simulink model "rti1401_program_controls_2018"  (R2017b)
settings: Solver=ode1  StartTime=0.0  StopTime=Inf  FixedStep=0.001  RelTol=1e-3  EnableMultiTasking=on
PreLoadFcn:
  | dataCar
  | load_vars
  | structAero
  | structEstimPar
  | structSensors
  | structSettings
PostLoadFcn:
  | , if any(exist('dsrtsu_mdlpostloadfcn', 'file') == [2, 3, 6]), try dsrtsu_mdlpostloadfcn('Execute', bdroot); catch fprintf('Error in PostLoadFcn (dsrtsu_mdlpostloadfcn) for model "%s":\n %s\n', bdroot, lasterr); end, end,
InitFcn:
  | dataCar
  | load_vars
  | structAero
  | structEstimPar
  | structSensors
  | structSettings
StartFcn:
  | dataCar
  | load_vars
  | structAero
  | structEstimPar
  | structSensors
  | structSettings
values from neighbouring files (symbols this model uses):
  Throttle_limits = [0.15, 0.90, 0.16, 0.92]    [load_vars.m]
undefined symbols (not defined in the file or in its folder): car, sensors, tau
libraries: rtican x44, hdlsllib x32, simulink x8, rti1401lib_II_base x1
(part 10 of 11)

== system rti1401_program_controls_2018/Processor/Decisive Logic Block ==
  TorqueController : Inport
  rpmController : Inport  Port=2
  TorqueBypass : Inport  Port=3
  rpmBypass : Inport  Port=4
  Settings : Inport  Port=5
  MATLAB Function : MATLAB Function  TreatAsAtomicUnit=on
  Torques : Outport
  rpmRef : Outport  Port=2
  wires:
  TorqueController/1 -> MATLAB Function/1(torqueController)
  rpmController/1 -> MATLAB Function/2(rpmController)
  TorqueBypass/1 -> MATLAB Function/3(torqueBypass)
  rpmBypass/1 -> MATLAB Function/4(rpmBypass)
  MATLAB Function/2(rpmRef) -> rpmRef/1
  Settings/1 -> MATLAB Function/5(settings)
  MATLAB Function/1(torques) -> Torques/1

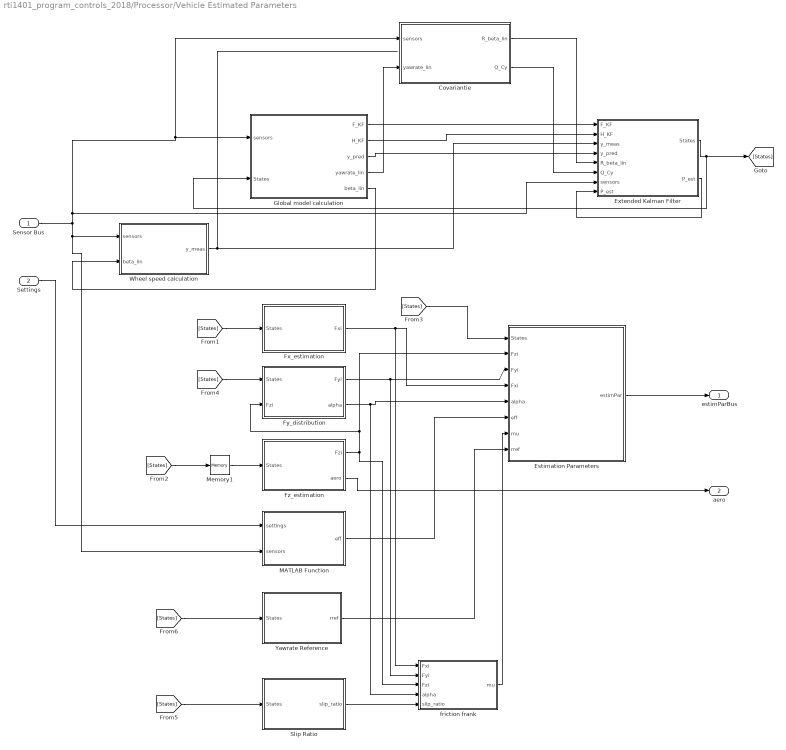
== system rti1401_program_controls_2018/Processor/Vehicle Estimated Parameters ==
  Sensor Bus : Inport
  Settings : Inport  Port=2
  Covariantie : MATLAB Function  TreatAsAtomicUnit=on
  Estimation Parameters : MATLAB Function  TreatAsAtomicUnit=on
  Extended Kalman Filter : MATLAB Function  TreatAsAtomicUnit=on
  Fx_estimation : MATLAB Function  TreatAsAtomicUnit=on
  Fy_distribution : MATLAB Function  TreatAsAtomicUnit=on
  Fz_estimation : MATLAB Function  TreatAsAtomicUnit=on
  Global model calculation : MATLAB Function  TreatAsAtomicUnit=on
  MATLAB Function : MATLAB Function  TreatAsAtomicUnit=on
  Memory1 : Memory
  Slip Ratio : MATLAB Function  TreatAsAtomicUnit=on
  Wheel speed calculation : MATLAB Function  TreatAsAtomicUnit=on
  Yawrate Reference : MATLAB Function  TreatAsAtomicUnit=on
  "friction frank  " : MATLAB Function  TreatAsAtomicUnit=on
  estimParBus : Outport
  aero : Outport  Port=2
  wires:
  Global model calculation/1(F_KF) -> Extended Kalman Filter/1(F_KF)
  Global model calculation/2(H_KF) -> Extended Kalman Filter/2(H_KF)
  Global model calculation/4(yawrate_lin) -> Covariantie/2(yawrate_lin)
  Wheel speed calculation/1(y_meas) -> Extended Kalman Filter/3(y_meas)
  Global model calculation/5(beta_lin) -> Wheel speed calculation/2(beta_lin)
  Covariantie/2(Q_Cy) -> Extended Kalman Filter/6(Q_Cy)
  Covariantie/1(R_beta_lin) -> Extended Kalman Filter/5(R_beta_lin)
  Extended Kalman Filter/1(States) -> [States], Global model calculation/2(States)
  Global model calculation/3(y_pred) -> Extended Kalman Filter/4(y_pred)
  Extended Kalman Filter/2(P_est) -> Extended Kalman Filter/8("P_est ")
  Estimation Parameters/1(estimPar) -> estimParBus/1
  [States] -> Fx_estimation/1(States)
  Memory1/1 -> Fz_estimation/1(States)
  [States] -> Memory1/1
  [States] -> Estimation Parameters/1(States)
  Fx_estimation/1(Fxi) -> "friction frank  "/1(Fxi), Estimation Parameters/4(Fxi)
  Fy_distribution/1(Fyi) -> "friction frank  "/2(Fyi), Estimation Parameters/3(Fyi)
  Fy_distribution/2(alpha) -> "friction frank  "/4(alpha), Estimation Parameters/5(alpha)
  [States] -> Fy_distribution/1(States)
  Fz_estimation/1(Fzi) -> "friction frank  "/3(Fzi), Fy_distribution/2(Fzi), Estimation Parameters/2(Fzi)
  Settings/1 -> MATLAB Function/1(settings)
  MATLAB Function/1(eff) -> Estimation Parameters/6(eff)
  Sensor Bus/1 -> Extended Kalman Filter/7(sensors), Covariantie/1(sensors), Global model calculation/1(sensors), MATLAB Function/2(sensors), Wheel speed calculation/1(sensors)
  "friction frank  "/1(mu) -> Estimation Parameters/7(mu)
  Slip Ratio/1(slip_ratio) -> "friction frank  "/5(slip_ratio)
  [States] -> Slip Ratio/1(States)
  Fz_estimation/2(aero) -> aero/1
  [States] -> Yawrate Reference/1(States)
  Yawrate Reference/1(rref) -> Estimation Parameters/8(rref)

== system rti1401_program_controls_2018/RTI Data/RTI Data Store ==
  RTI Data Store : Subsystem  mask(RTI_DATA_STORE){}
      mask help:
      | RTI Data Store Block. This block is used by RTI to store internal model dependent data. Deleting this block will result in data loss.
      |
      | NEVER DELETE, COPY, OR MODIFY THIS BLOCK!
      mask Help:
      | RTI Data Store Block. This block is used by RTI to store internal model dependent data. Deleting this block will result in data loss.
      | 
      | NEVER DELETE, COPY, OR MODIFY THIS BLOCK!
      mask Display: text(0.5, 0.5, ' ', 'HorizontalAlignment', 'center');

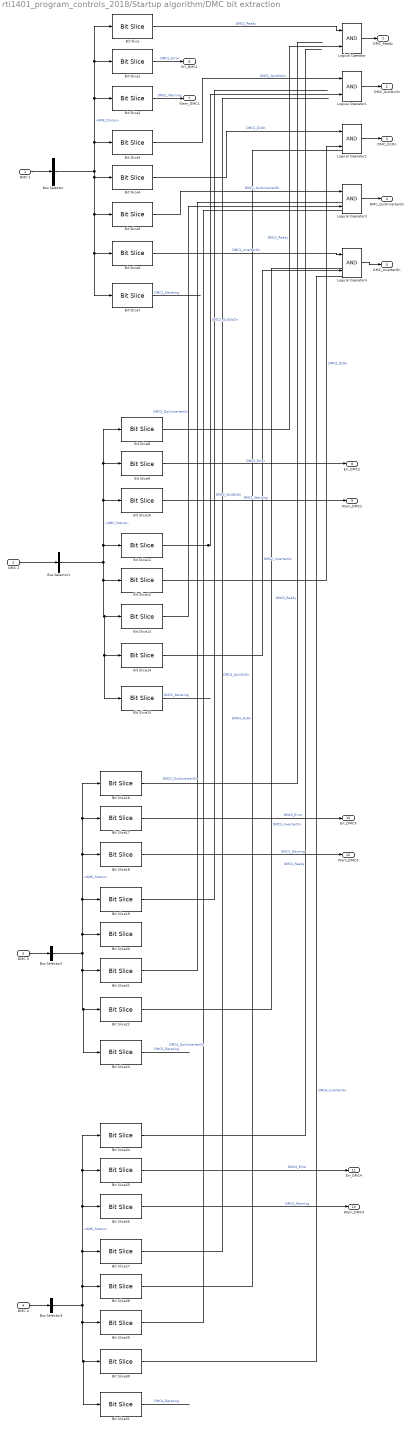
== system rti1401_program_controls_2018/Startup algorithm/DMC bit extraction ==
  DMC 1 : Inport
  DMC 2 : Inport  Port=2
  DMC 3 : Inport  Port=3
  DMC 4 : Inport  Port=4
  Bit Slice{,8,16,24} (4 alike) : hdlsllib/Logic and Bit Operations/Bit Slice  lidx=8  ridx=8
  Bit Slice{1,9,17,25} (4 alike) : hdlsllib/Logic and Bit Operations/Bit Slice  lidx=9  ridx=9
  Bit Slice{2,10,18,26} (4 alike) : hdlsllib/Logic and Bit Operations/Bit Slice  lidx=10  ridx=10
  Bit Slice{3,11,19,27} (4 alike) : hdlsllib/Logic and Bit Operations/Bit Slice  lidx=11  ridx=11
  Bit Slice{4,12,20,28} (4 alike) : hdlsllib/Logic and Bit Operations/Bit Slice  lidx=12  ridx=12
  Bit Slice{5,13,21,29} (4 alike) : hdlsllib/Logic and Bit Operations/Bit Slice  lidx=13  ridx=13
  Bit Slice{6,14,22,30} (4 alike) : hdlsllib/Logic and Bit Operations/Bit Slice  lidx=14  ridx=14
  Bit Slice{7,15,23,31} (4 alike) : hdlsllib/Logic and Bit Operations/Bit Slice  lidx=15  ridx=15
  Bus Selector{,1..3} (4 alike) : BusSelector  OutputSignals=AMK_Status
  Logical Operator{,1..4} (5 alike) : Logic  AllPortsSameDT=off  OutDataTypeStr=boolean
  DMC_Ready : Outport
  DMC_QuitDcOn : Outport  Port=2
  DMC_DcOn : Outport  Port=3
  DMC_QuitInverterOn : Outport  Port=4
  DMC_InverterOn : Outport  Port=5
  Err_DMC1 : Outport  Port=6
  Warn_DMC1 : Outport  Port=7
  Err_DMC2 : Outport  Port=8
  Warn_DMC2 : Outport  Port=9
  Err_DMC3 : Outport  Port=10
  Err_DMC4 : Outport  Port=11
  Warn_DMC3 : Outport  Port=12
  Warn_DMC4 : Outport  Port=13
  wires:
  DMC 4/1 -> Bus Selector3/1
  DMC 3/1 -> Bus Selector2/1
  DMC 1/1 -> Bus Selector/1
  DMC 2/1 -> Bus Selector1/1
  Bus Selector/1 -> Bit Slice7/1, Bit Slice6/1, Bit Slice5/1, Bit Slice4/1, Bit Slice/1, Bit Slice1/1, Bit Slice2/1, Bit Slice3/1  "<AMK_Status>"
  Bit Slice/1 -> Logical Operator/1  "DMC1_Ready"
  Bit Slice1/1 -> Err_DMC1/1  "DMC1_Error"
  Bit Slice2/1 -> Warn_DMC1/1  "DMC1_Warning"
  Bit Slice3/1 -> Logical Operator1/1  "DMC1_QuitDcOn"
  Bit Slice4/1 -> Logical Operator2/1  "DMC1_DcOn"
  Bit Slice5/1 -> Logical Operator3/1  "DMC1_QuitInverterOn"
  Bit Slice6/1 -> Logical Operator4/1  "DMC1_InverterOn"
  Bit Slice7/1 -> ?  "DMC1_Derating"
  Bus Selector1/1 -> Bit Slice15/1, Bit Slice14/1, Bit Slice13/1, Bit Slice12/1, Bit Slice8/1, Bit Slice9/1, Bit Slice10/1, Bit Slice11/1  "<AMK_Status>"
  Bit Slice8/1 -> Logical Operator/2  "DMC2_Ready"
  Bit Slice9/1 -> Err_DMC2/1  "DMC2_Error"
  Bit Slice10/1 -> Warn_DMC2/1  "DMC2_Warning"
  Bit Slice11/1 -> Logical Operator1/2  "DMC2_QuitDcOn"
  Bit Slice12/1 -> Logical Operator2/2  "DMC2_DcOn"
  Bit Slice13/1 -> Logical Operator3/2  "DMC2_QuitInverterOn"
  Bit Slice14/1 -> Logical Operator4/2  "DMC2_InverterOn"
  Bit Slice15/1 -> ?  "DMC2_Derating"
  Bus Selector2/1 -> Bit Slice16/1, Bit Slice17/1, Bit Slice18/1, Bit Slice19/1, Bit Slice20/1, Bit Slice23/1, Bit Slice22/1, Bit Slice21/1  "<AMK_Status>"
  Bit Slice16/1 -> ?  "DMC3_Ready"
  Bit Slice17/1 -> Err_DMC3/1  "DMC3_Error"
  Bit Slice18/1 -> Warn_DMC3/1  "DMC3_Warning"
  Bit Slice19/1 -> ?  "DMC3_QuitDcOn"
  Bit Slice21/1 -> ?  "DMC3_QuitInverterOn"
  Bit Slice22/1 -> ?  "DMC3_InverterOn"
  Bit Slice23/1 -> ?  "DMC3_Derating"
  Bus Selector3/1 -> Bit Slice24/1, Bit Slice25/1, Bit Slice26/1, Bit Slice27/1, Bit Slice28/1, Bit Slice31/1, Bit Slice30/1, Bit Slice29/1  "<AMK_Status>"
  Bit Slice24/1 -> ?  "DMC4_Ready"
  Bit Slice25/1 -> Err_DMC4/1  "DMC4_Error"
  Bit Slice26/1 -> Warn_DMC4/1  "DMC4_Warning"
  Bit Slice27/1 -> ?  "DMC4_QuitDcOn"
  Bit Slice28/1 -> ?  "DMC4_DcOn"
  Bit Slice29/1 -> ?  "DMC4_QuitInverterOn"
  Bit Slice30/1 -> ?  "DMC4_InverterOn"
  Bit Slice31/1 -> ?  "DMC4_Derating"
  Logical Operator/1 -> DMC_Ready/1
  Logical Operator1/1 -> DMC_QuitDcOn/1
  Logical Operator2/1 -> DMC_DcOn/1
  Logical Operator3/1 -> DMC_QuitInverterOn/1
  Logical Operator4/1 -> DMC_InverterOn/1

== system rti1401_program_controls_2018/Startup algorithm/Merge_Controlword ==
  Control_in : Inport
  DcOn : Inport  Port=2
  Enable : Inport  Port=3
  InverterOn : Inport  Port=4
  ErrorReset : Inport  Port=5
  Bus Creator : BusCreator  Inputs=4
  If CTRL = Null : MATLAB Function  TreatAsAtomicUnit=on
  Control : Outport
  wires:
  Enable/1 -> If CTRL = Null/3(En_in)
  InverterOn/1 -> If CTRL = Null/4(Inv_in)
  DcOn/1 -> If CTRL = Null/2(Dc_in)
  Control_in/1 -> If CTRL = Null/1(Ctrl_in)
  If CTRL = Null/1(DcOn) -> Bus Creator/1
  If CTRL = Null/2(Enable) -> Bus Creator/2
  If CTRL = Null/3(InverterOn) -> Bus Creator/3
  Bus Creator/1 -> Control/1  "Controlbits"
  ErrorReset/1 -> Bus Creator/4  "ErrorReset"

== system rti1401_program_controls_2018/Processor/Control Systems/Distributor ==
  sensors : Inport
  settings : Inport  Port=2
  estimPar : Inport  Port=3
  Mz : Inport  Port=4
  Aero : Inport  Port=5
  MATLAB Function : MATLAB Function  TreatAsAtomicUnit=on
  Mux : Mux
  To Workspace : ToWorkspace  VariableName=Fdes  SaveFormat=Timeseries  SampleTime=-1
  To Workspace1 : ToWorkspace  VariableName=Fxmax  SaveFormat=Timeseries  SampleTime=-1
  To Workspace2 : ToWorkspace  VariableName=MdesFdesFxmaxFx  SaveFormat=Timeseries  SampleTime=-1
  To Workspace4 : ToWorkspace  VariableName=Fx  SaveFormat=Timeseries  SampleTime=-1
  Torque/Brake analyzer : Subsystem
  torqueDistribution : Outport
  slipSet : Outport  Port=2
  wires:
  MATLAB Function/1(torqueDistribution) -> torqueDistribution/1
  sensors/1 -> Torque/Brake analyzer/1(sensors), MATLAB Function/1(sensors)
  settings/1 -> Torque/Brake analyzer/2(settings), MATLAB Function/2(settings)
  estimPar/1 -> Torque/Brake analyzer/3(estimPar), MATLAB Function/3(estimPar)
  Mz/1 -> Mux/1, MATLAB Function/4(Mz)
  MATLAB Function/2(slipSet) -> slipSet/1
  MATLAB Function/3(Fdes) -> Mux/2, To Workspace/1
  Mux/1 -> To Workspace2/1
  MATLAB Function/5(Fx) -> To Workspace4/1, Mux/4
  MATLAB Function/4(Fxmax) -> To Workspace1/1, Mux/3
  Torque/Brake analyzer/1(Fdes) -> MATLAB Function/5("Fdes ")
  Aero/1 -> Torque/Brake analyzer/4(Aero)

== system rti1401_program_controls_2018/Processor/Control Systems/Power Checker ==
  Sensors : Inport
  Settings : Inport  Port=2
  "estimPar  " : Inport  Port=3
  unchecked torque : Inport  Port=4
  Power checker : MATLAB Function  TreatAsAtomicUnit=on
  CheckedTorque : Outport
  wires:
  Sensors/1 -> Power checker/1(sensors)
  Settings/1 -> Power checker/2(settings)
  Power checker/1(CheckedTorque) -> CheckedTorque/1
  "estimPar  "/1 -> Power checker/3(estimPar)
  unchecked torque/1 -> Power checker/4(UncheckedTorque)

== system rti1401_program_controls_2018/RTI Data/RTI Data Store/RTI Data Store ==
  RTI Data Store : Subsystem  mask(RTI_DATA_STORE){}
      mask help:
      | RTI Data Store Block. This block is used by RTI to store internal model dependent data. Deleting this block will result in data loss.
      |
      | NEVER DELETE, COPY, OR MODIFY THIS BLOCK!
      mask Help:
      | RTI Data Store Block. This block is used by RTI to store internal model dependent data. Deleting this block will result in data loss.
      | 
      | NEVER DELETE, COPY, OR MODIFY THIS BLOCK!
      mask Display: text(0.5, 0.5, ' ', 'HorizontalAlignment', 'center');

== system rti1401_program_controls_2018/Processor/Control Systems/Distributor/Torque//Brake analyzer ==
  sensors : Inport
  settings : Inport  Port=2
  estimPar : Inport  Port=3
  Aero : Inport  Port=4
  MATLAB Function1 : MATLAB Function  TreatAsAtomicUnit=on
  Fdes : Outport
  wires:
  MATLAB Function1/1(Fdes) -> Fdes/1
  sensors/1 -> MATLAB Function1/1(sensors)
  settings/1 -> MATLAB Function1/2(settings)
  estimPar/1 -> MATLAB Function1/3(estimPar)
  Aero/1 -> MATLAB Function1/4(aero)

== system rti1401_program_controls_2018/RTI Data/RTI Data Store/RTI Data Store/RTI Data Store ==
  RTI Data Store : Subsystem  mask(RTI_DATA_STORE){}
      mask help:
      | RTI Data Store Block. This block is used by RTI to store internal model dependent data. Deleting this block will result in data loss.
      |
      | NEVER DELETE, COPY, OR MODIFY THIS BLOCK!
      mask Help:
      | RTI Data Store Block. This block is used by RTI to store internal model dependent data. Deleting this block will result in data loss.
      | 
      | NEVER DELETE, COPY, OR MODIFY THIS BLOCK!
      mask Display: text(0.5, 0.5, ' ', 'HorizontalAlignment', 'center');

== system rti1401_program_controls_2018/RTI Data/RTI Data Store/RTI Data Store/RTI Data Store/RTI Data Store ==

== matlab function rti1401_program_controls_2018/Inputs/Preprocessor/MATLAB Function ==
  data: Throttle1 input; error output; Throttle2 input; limits input; throttle output
function [error,throttle]= ThrottleSensorPreprocessor(Throttle1, Throttle2, limits)
% Variables
lowerlim1 = limits(1);
upperlim1 = limits(2);
lowerlim2 = limits(3);
upperlim2 = limits(4);

% Throttle sensor 1

if Throttle1<lowerlim1
    y1=0;
elseif Throttle1>upperlim1
    y1=1;
else
   y1=Throttle1; %%schalen???
end

%Throttle sensor 2

if Throttle2<lowerlim2
    y2=0;
elseif Throttle2>upperlim2
    y2=1;
else
   y2=Throttle2; %%schalen???
end


% Error
if abs(Throttle1-Throttle2) > 0.10
    error = 1;
    throttle = 0;
else
    error = 0;
    throttle = double((y1+y2)/2);
end

== matlab function rti1401_program_controls_2018/Outputs/Splitter ==
  data: Torques input; torqueFL_Pos output; torqueFL_Neg output; wheelspeedFL output; torqueFR_Pos output; torqueFR_Neg output; wheelspeedFR output; torqueRL_Pos output; torqueRL_Neg output; wheelspeedRL output; torqueRR_Pos output; torqueRR_Neg output; wheelspeedRR output; status input; car parameter
function [torqueFL_Pos, torqueFL_Neg, wheelspeedFL, ...
    torqueFR_Pos, torqueFR_Neg, wheelspeedFR, ...
    torqueRL_Pos, torqueRL_Neg, wheelspeedRL, ...
    torqueRR_Pos, torqueRR_Neg, wheelspeedRR]= Splitter(Torques, status, car)

inversetorque = car.motor.Tmax;

if (status == 4)

    if Torques(1) >= 0
        torqueFL_Pos = int16(Torques(1)*1000);
        torqueFL_Neg = int16(-inversetorque(1)*1000);
        wheelspeedFL = int16(500);
    else
        torqueFL_Pos = int16(inversetorque(1)*1000);
        torqueFL_Neg = int16(Torques(1)*1000);
        wheelspeedFL = int16(0);
    end

    if Torques(2) >= 0
        torqueFR_Pos = int16(Torques(2)*1000);
        torqueFR_Neg = int16(-inversetorque(2)*1000);
        wheelspeedFR = int16(500);
    else
        torqueFR_Pos = int16(inversetorque(2)*1000);
        torqueFR_Neg = int16(Torques(2)*1000);
        wheelspeedFR = int16(0);
    end

    if Torques(3) >= 0
        torqueRL_Pos = int16(Torques(3)*1000);
        torqueRL_Neg = int16(-inversetorque(3)*1000);
        wheelspeedRL = int16(500);
    else
        torqueRL_Pos = int16(inversetorque(3)*1000);
        torqueRL_Neg = int16(Torques(3)*1000);
        wheelspeedRL = int16(0);
    end

    if Torques(4) >= 0
        torqueRR_Pos = int16(Torques(4)*1000);
        torqueRR_Neg = int16(-inversetorque(4)*1000);
        wheelspeedRR = int16(500);
    else
        torqueRR_Pos = int16(inversetorque(4)*1000);
        torqueRR_Neg = int16(Torques(4)*1000);
        wheelspeedRR = int16(0);
    end
else
    torqueFL_Pos = int16(0);
    torqueFL_Neg = int16(0);
    wheelspeedFL = int16(0);
    torqueFR_Pos = int16(0);
    torqueFR_Neg = int16(0);
    wheelspeedFR = int16(0);
    torqueRL_Pos = int16(0);
    torqueRL_Neg = int16(0);
    wheelspeedRL = int16(0);
    torqueRR_Pos = int16(0);
    torqueRR_Neg = int16(0);
    wheelspeedRR = int16(0);
end

== matlab function rti1401_program_controls_2018/Inputs/Preprocessor/Throttle1 perc ==
  data: u input; y output
function y = percentage(u)
y = ((1024 - double(u)) - 74) / 380;

== matlab function rti1401_program_controls_2018/Inputs/Preprocessor/Throttle2 perc off ==
  data: u input; y output
function y = percoff(u)
y = (1024 - double(u) - 374) / 420;

== matlab function rti1401_program_controls_2018/Inputs/Preprocessor/Acc conversion ==
  data: x input; y input; z input; AccX output; AccY output; AccZ output
function [AccX,AccY,AccZ] = AccConv(x,y,z)
AccX = x*9.81;
AccY = y*9.81;
AccZ = z*9.81;

== matlab function rti1401_program_controls_2018/Inputs/Preprocessor/YR//RR conversion ==
  data: y input; r input; Y output; R output
function [Y,R] = YRRR(y,r)
Y = y*10*2*pi;
R = r*10*2*pi;

== matlab function rti1401_program_controls_2018/Inputs/Preprocessor/Steering conv ==
  data: u input; Steering output
function Steering = steeringangle(u)
t = double(u);
Steering = 1 * t; %TODO: conversion factor, output = rack travel in mm

== matlab function rti1401_program_controls_2018/Inputs/EnergyMeter/parseCurrent  ==
  data: Mux input; current output; status input; messageNr input; valueHighest input; valueMidHigh input; valueMidLow input; valueLowest input
function current = value(Mux,status,messageNr,valueHighest,valueMidHigh, valueMidLow, valueLowest)
%    format hex;
   
  
    value = [valueLowest, valueMidLow, valueMidHigh, valueHighest];
    value = typecast(value, 'uint32');
    current=uint32(0);
    %0 is current
%     disp (Mux);
%     disp (status);
%     disp (messageNr);
%     disp (valueHigh);
%     disp (valueLow);
%     value = [valueHigh,valueLow];
%     disp (value);
    if Mux==0
        if status==0
            %status ok
            current = value %swapbytes(typecast(value,'uint32'));%current in mA
        else
        end
    end
%     disp (current);
%     format long;
%     disp (current);
end

== matlab function rti1401_program_controls_2018/Inputs/EnergyMeter/parseVoltage1 ==
  data: Mux input; voltage1 output; status input; messageNr input; valueHighest input; valueMidHigh input; valueMidLow input; valueLowest input
function voltage1 = value(Mux,status,messageNr,valueHighest,valueMidHigh,valueMidLow,valueLowest)
%    format hex;
    voltage1=uint32(0);
    %0 is current
%     disp (Mux);
%     disp (status);
%     disp (messageNr);
%     disp (valueHigh);
%     disp (valueLow);
    value = [valueLowest, valueMidLow, valueMidHigh, valueHighest];
    value = typecast(value, 'uint32');
%     disp (value);
    if Mux==1
        if status==0
            %status ok
            voltage1 = value;
        else
        end
    end
%     disp (current);
%     format long;
%     disp (current);
end

== matlab function rti1401_program_controls_2018/Inputs/EnergyMeter/parseVoltage3 ==
  data: Mux input; voltage3 output; status input; messageNr input; valueHighest input; valueMidHigh input; valueMidLow input; valueLowest input
function voltage3 = value(Mux,status,messageNr,valueHighest,valueMidHigh,valueMidLow,valueLowest)
%    format hex;
   
    voltage3=uint32(0);
    %0 is current
%     disp (Mux);
%     disp (status);
%     disp (messageNr);
%     disp (valueHigh);
%     disp (valueLow);
    value = [valueLowest, valueMidLow, valueMidHigh, valueHighest];
    value = typecast(value, 'uint32');
%     disp (value);
    if Mux==3
        if status==0
            %status ok
            voltage3 = value;
        else
        end
    end
%     disp (current);
%     format long;
%     disp (current);
end

== matlab function rti1401_program_controls_2018/Inputs/EnergyMeter/parseTemperature ==
  data: Mux input; temperature output; status input; messageNr input; valueHighest input; valueMidHigh input; valueMidLow input; valueLowest input
function temperature = value(Mux,status,messageNr,valueHighest,valueMidHigh,valueMidLow,valueLowest)
%    format hex;
    
    temperature=uint32(0);
    %0 is current
%     disp (Mux);
%     disp (status);
%     disp (messageNr);
%     disp (valueHigh);
%     disp (valueLow);
    value = [valueLowest, valueMidLow, valueMidHigh, valueHighest];
    value = typecast(value, 'uint32');
%     disp (value);
    if Mux==4
        if status==0
            %status ok
            temperature =value;
        else
        end
    end
%     disp (current);
%     format long;
%     disp (current);
end

== matlab function rti1401_program_controls_2018/Inputs/EnergyMeter/parseEnergy ==
  data: Mux input; energy output; status input; messageNr input; valueHighest input; valueMidHigh input; valueMidLow input; valueLowest input
function energy = value(Mux,status,messageNr,valueHighest,valueMidHigh,valueMidLow,valueLowest)
%    format hex;
    
    energy= uint32(0);
    %0 is current
%     disp (Mux);
%     disp (status);
%     disp (messageNr);
%     disp (valueHigh);
%     disp (valueLow);
    value = [valueLowest, valueMidLow, valueMidHigh, valueHighest];
    value = typecast(value, 'uint32');
%     disp (value);
    if Mux==5
        if status==0
            %status ok
            energy =value;
        else
        end
    end
%     disp (current);
%     format long;
%     disp (current);
end

== matlab function rti1401_program_controls_2018/Inputs/EnergyMeter/MATLAB Function ==
  data: muxByte input; response output; response0 input; response1 input; response2 input; response3 input; response4 input; response5 input; response6 input
function response = response(muxByte,response0, response1,response2,response3,response4,response5,response6)
    error = uint8(255);
    size = zeros(1,7);
    response = uint8(size);
    if (muxByte >= 128 && muxByte < 144)
       %error/log data
       if (muxByte < 130) % 0x82
          response(1) = error;
       end
       if (muxByte == 130||muxByte == 131) %response on overal logdata, 0x82 en 0x83
           response = [response0, response1, response2, response3, response4, response5, response6];
       end
    end
    if (muxByte >=144 && muxByte < 160)
       %can id 
       switch muxByte
           case 144
           case 145
           case 146
           case 147
           case 148
           case 149
           case 150
           case 151
           case 157
           case 159
           otherwise
               response(1) = error;
       end               
    end
    if (muxByte >=160 && muxByte < 176)
       %config result
       %cases zoals bij 90
       %default
       response(1) = error;
    end
    if (muxByte >=176 && muxByte < 192)
        %set en get commands
        %B0 - B6, B9 - BC
        response(1) = error;
    end
    if (muxByte == 255)
        response(1) = error;
    end
end

== matlab function rti1401_program_controls_2018/Setup/MATLAB Function ==
  data: messageByte0 output; messageByte1 output; messageByte2 output; messageByte3 output; messageByte4 output; messageByte5 output; messageByte6 output; messageByte7 output; progress output; initialProgress input
function [messageByte0,messageByte1,messageByte2,messageByte3, messageByte4, messageByte5, messageByte6,messageByte7,progress] = setup(initialProgress)
    progress = initialProgress;
    messageValue = uint8(zeros(1,8));
    if (progress<5)
        if(progress==0)
            messageValue(1) = uint8(52); %0x34 set_mode --> stop
            messageValue(2:8)= uint8(zeros(1,7));
            progress=1;
        elseif(progress==1)
            messageValue(1) = uint8(33); %0x21 set configuration of U1
            messageValue(2) = uint8(2); %0x02 cyclisch && big endian
            messageValue(3:4) = uint8([0 50]); %50ms 
            messageValue(5:8) = zeros(1,4);
            progress=2;
        elseif(progress==2)
            messageValue(1) = uint8(37); %0x25 set configuration of W
            messageValue(2) = uint8(2); %0x02 cyclisch && big endian
            messageValue(3:4) = uint8([0 50]); %50ms 
            messageValue(5:8) = zeros(1,4);
            progress = 3;
        elseif(progress ==3)
            messageValue(1) = uint8(38); %0x26 set configuration of As
            messageValue(2) = uint8(2); %0x02 cyclisch && big endian
            messageValue(3:4) = uint8([0 50]); %50ms 
            messageValue(5:8) = zeros(1,4);
            progress = 4;
        elseif (progress ==4)
            messageValue(1) = uint8(52); %0x34 set_mode--> start
            messageValue(2:3) = uint8(ones(1,2));
            messageValue(4:8) = zeros(1,5);
            progress=5;
        end
    end
    messageByte0 = messageValue(1);
    messageByte1 = messageValue(2);
    messageByte2 = messageValue(3);
    messageByte3 = messageValue(4);
    messageByte4 = messageValue(5);
    messageByte5 = messageValue(6);
    messageByte6 = messageValue(7);
    messageByte7 = messageValue(8);
end

== matlab function rti1401_program_controls_2018/Processor/Lode Torque Conversion Block ==
  data: currentFL input; torqueFL output; currentFR input; currentRL input; currentRR input; torqueFR output; torqueRL output; torqueRR output
function [torqueFL,torqueFR,torqueRL,torqueRR] = torqueConversion(currentFL,currentFR,currentRL,currentRR)
currentFL = double(currentFL);
currentFR = double(currentFR);
currentRL = double(currentRL);
currentRR = double(currentRR);

ID110 = 107.2; %Converter peak current (from Ipex Pro)

%4.1837 = Nominal Current/Nominal Torque = 41A/9.8Nm (from AMK data sheet)
%--> Ook geldig voor anno 2018!!

IqFL = currentFL * ID110 / 16384; %I_q (AMK manual P65)
torqueFL = IqFL / 4.1837; %T (AMK manual P65)

IqFR = currentFR * ID110 / 16384; %I_q (AMK manual P65)
torqueFR = IqFR / 4.1837; %T (AMK manual P65)

IqRL = currentRL * ID110 / 16384; %I_q (AMK manual P65)
torqueRL = IqRL / 4.1837; %T (AMK manual P65)

IqRR = currentRR * ID110 / 16384; %I_q (AMK manual P65)
torqueRR = IqRR / 4.1837; %T (AMK manual P65)

== matlab function rti1401_program_controls_2018/Inputs/EnergyMeter/parseVoltage2 ==
  data: Mux input; voltage2 output; status input; messageNr input; valueHighest input; valueMidHigh input; valueMidLow input; valueLowest input
function voltage2 = value(Mux,status,messageNr,valueHighest,valueMidHigh,valueMidLow,valueLowest)
%    format hex;
    
    voltage2=uint32(0);
    %0 is current
%     disp (Mux);
%     disp (status);
%     disp (messageNr);
%     disp (valueHigh);
%     disp (valueLow);
    value = [valueLowest, valueMidLow, valueMidHigh, valueHighest];
    value = typecast(value, 'uint32');
%     disp (value);
    if Mux==2
        if status==0
            %status ok
            voltage2 = value;
        else
        end
    end
%     disp (current);
%     format long;
%     disp (current);
end

== matlab function rti1401_program_controls_2018/Inputs/EnergyMeter/parseAs ==
  data: Mux input; ampereSeconde output; status input; messageNr input; valueHighest input; valueMidHigh input; valueMidLow input; valueLowest input
function ampereSeconde = value(Mux,status,messageNr,valueHighest,valueMidHigh,valueMidLow,valueLowest)
%    format hex;
    ampereSeconde=uint32(6);
    %0 is current
%     disp (Mux);
%     disp (status);
%     disp (messageNr);
%     disp (valueHigh);
%     disp (valueLow);
    value = [valueLowest, valueMidLow, valueMidHigh, valueHighest];
    value = typecast(value, 'uint32');
%     disp (value);
    if Mux==3
        if status==0
            %status ok
            ampereSeconde = value;
        else
        end
    end
%     disp (current);
%     format long;
%     disp (current);
end

== matlab function rti1401_program_controls_2018/Inputs/EnergyMeter/parseWh ==
  data: Mux input; wattHour output; status input; messageNr input; valueHighest input; valueMidHigh input; valueMidLow input; valueLowest input
function wattHour = value(Mux,status,messageNr,valueHighest,valueMidHigh,valueMidLow,valueLowest)
%    format hex;
 
    wattHour=uint32(0);
    %0 is current
%     disp (Mux);
%     disp (status);
%     disp (messageNr);
%     disp (valueHigh);
%     disp (valueLow);
    value = [valueLowest, valueMidLow, valueMidHigh, valueHighest];
    value = typecast(value, 'uint32');
%     disp (value);
    if Mux==7
        if status==0
            %status ok
            wattHour = value;
        else
        end
    end
%     disp (current);
%     format long;
%     disp (current);
end

== stateflow chart rti1401_program_controls_2018/Startup algorithm/Startup ==
  state LVOn
    entry: AMK_Control = 1;
    entry: BMS_START= 1;
    entry: AMK_DcOn = 0;
    entry: AMK_Enable = 0;
    entry: AMK_InverterOn = 0;
    entry: Status = 0;
  state SystemReady
    entry: BMS_START = 1;
    entry: Status = 1;
  state SwitchDCOn
    entry: Status = 2;
    entry: AMK_DcOn = 1;
  state PreparingToDrive
    entry: AMK_Enable = 1;
    entry: AMK_InverterOn = 1;
    entry: RTDS = true;
    entry: Status = 3;
  state Running
    entry: Status = 4;
    entry: RTDS = false;
  SystemReady -> LVOn [order 2] : [Stop==1]
  (default) -> LVOn
  LVOn -> SystemReady : [AMK_Systemready == 1 && Stop==0]
  Running -> LVOn : [Stop == 1]
  SystemReady -> SwitchDCOn [order 1] : [Start==1]
  PreparingToDrive -> LVOn [order 2] : [Stop ==1]
  SwitchDCOn -> LVOn [order 2] : [Stop == 1]
  SwitchDCOn -> PreparingToDrive [order 1] : [QuitDcOn==1 && DcOn==1]
  PreparingToDrive -> Running [order 1] : [InverterOn==1 && QuitInverterOn==1]
  data: AMK_Systemready input; BMS_HV input; AMK_Control output; AMK_DcOn output; AMK_Enable output; AMK_InverterOn output; BMS_START output; RTDS output; Status output; QuitDcOn input; DcOn input; InverterOn input; QuitInverterOn input; Start input; Stop input

== matlab function rti1401_program_controls_2018/Inputs/Preprocessor/Brake 1 perc  ==
  data: u input; y output
function y = percentage(u)
y = u/65536;

== matlab function rti1401_program_controls_2018/Inputs/Preprocessor/Brake 2 perc  ==
  data: u input; y output
function y = percentage(u)
y = u/65536;

== matlab function rti1401_program_controls_2018/Startup algorithm/Merge_Controlword/If CTRL = Null ==
  data: Ctrl_in input; DcOn output; Dc_in input; En_in input; Inv_in input; Enable output; InverterOn output
function [DcOn, Enable, InverterOn] = fcn(Ctrl_in, Dc_in, En_in, Inv_in)
%#codegen

if (Ctrl_in==0)
    DcOn = false;
    Enable = false;
    InverterOn = false;
else
    DcOn = logical(Dc_in);
    Enable = logical(En_in);
    InverterOn = logical(Inv_in);
end

== matlab function rti1401_program_controls_2018/Processor/Breyne Pedal Mapping ==
  data: throttle input; throttle_out output; regen input; brake_out output
function [throttle_out, brake_out] = pedalmapping(throttle, regen)

%Pedal mapping: partially regenarative braking (parabolic), partially positive 
%power (parabolic and linear)
%IMPORTANT: D = shape factor = relative y-value where parabolic switches to linear
% (between 0 and 1)
% LOW D = more linear
% HIGH D = more parabolic

D = double(0);

%%
regen = double(max(min(regen,30),0));
throttle_acc = double((throttle-regen)/(100-regen));
if throttle >= regen
    if throttle <= regen+(100-regen)*(2*D)/(1+D)
        if throttle == regen %iow if D==0
            throttle_out = double(0);
        else
            parab = (1+D)^2/(4*D)*throttle_acc^2;
            throttle_out = double(100*parab);
        end
    else 
        lin = (1+D)*throttle_acc-D;
        throttle_out = 100*lin;
    end
    brake_out = 0;
else
    if regen == 0
        brake_out = 0;
    else
        brake_out = double((-1/regen)*throttle^2+2*throttle-regen);
    end
    throttle_out = 0;
end

%% implausibility check
throttle_out = max(min(throttle_out,100),0);
brake_out = max(min(brake_out,100),0);

== matlab function rti1401_program_controls_2018/Outputs/Drives/Merge_bits ==
  data: AMK_bInverterOn input; AMK_Control output; AMK_bDcOn input; AMK_bEnable input; AMK_bErrorReset input
function AMK_Control = AMK_Control(AMK_bInverterOn, AMK_bDcOn, AMK_bEnable, AMK_bErrorReset)

AMK_bDcOn_shift = bitsll(uint8(AMK_bDcOn),1);               %shift DcOn bit 1 times to left
AMK_bEnable_shift = bitsll(uint8(AMK_bEnable),2);           %shift Enable bit 2 times to left
AMK_bErrorReset_shift = bitsll(uint8(AMK_bErrorReset),3);   %shift ErrorReset bit 3 times to left

AMK_Control = uint8(AMK_bInverterOn);                           %bit 0 is InvertOn bit
AMK_Control = bitor(AMK_Control,uint8(AMK_bDcOn_shift));        %bitwise OR AMK_Control with shifter DcOn bit
AMK_Control = bitor(AMK_Control,uint8(AMK_bEnable_shift));      %bitwise OR AMK_Control with shifted Enable bit
AMK_Control = bitor(AMK_Control,uint8(AMK_bErrorReset_shift));  %bitwise OR AMK_Control with shifted ErrorReset bit

== matlab function rti1401_program_controls_2018/Outputs/Drives/Merge_bits1 ==
  data: AMK_bInverterOn input; AMK_Control output; AMK_bDcOn input; AMK_bEnable input; AMK_bErrorReset input
function AMK_Control = AMK_Control(AMK_bInverterOn, AMK_bDcOn, AMK_bEnable, AMK_bErrorReset)

AMK_bDcOn_shift = bitsll(uint8(AMK_bDcOn),1);               %shift DcOn bit 1 times to left
AMK_bEnable_shift = bitsll(uint8(AMK_bEnable),2);           %shift Enable bit 2 times to left
AMK_bErrorReset_shift = bitsll(uint8(AMK_bErrorReset),3);   %shift ErrorReset bit 3 times to left

AMK_Control = uint8(AMK_bInverterOn);                           %bit 0 is InvertOn bit
AMK_Control = bitor(AMK_Control,uint8(AMK_bDcOn_shift));        %bitwise OR AMK_Control with shifter DcOn bit
AMK_Control = bitor(AMK_Control,uint8(AMK_bEnable_shift));      %bitwise OR AMK_Control with shifted Enable bit
AMK_Control = bitor(AMK_Control,uint8(AMK_bErrorReset_shift));  %bitwise OR AMK_Control with shifted ErrorReset bit

== matlab function rti1401_program_controls_2018/Outputs/Drives/Merge_bits2 ==
  data: AMK_bInverterOn input; AMK_Control output; AMK_bDcOn input; AMK_bEnable input; AMK_bErrorReset input
function AMK_Control = AMK_Control(AMK_bInverterOn, AMK_bDcOn, AMK_bEnable, AMK_bErrorReset)

AMK_bDcOn_shift = bitsll(uint8(AMK_bDcOn),1);               %shift DcOn bit 1 times to left
AMK_bEnable_shift = bitsll(uint8(AMK_bEnable),2);           %shift Enable bit 2 times to left
AMK_bErrorReset_shift = bitsll(uint8(AMK_bErrorReset),3);   %shift ErrorReset bit 3 times to left

AMK_Control = uint8(AMK_bInverterOn);                           %bit 0 is InvertOn bit
AMK_Control = bitor(AMK_Control,uint8(AMK_bDcOn_shift));        %bitwise OR AMK_Control with shifter DcOn bit
AMK_Control = bitor(AMK_Control,uint8(AMK_bEnable_shift));      %bitwise OR AMK_Control with shifted Enable bit
AMK_Control = bitor(AMK_Control,uint8(AMK_bErrorReset_shift));  %bitwise OR AMK_Control with shifted ErrorReset bit

== matlab function rti1401_program_controls_2018/Outputs/Drives/Merge_bits3 ==
  data: AMK_bInverterOn input; AMK_Control output; AMK_bDcOn input; AMK_bEnable input; AMK_bErrorReset input
function AMK_Control = AMK_Control(AMK_bInverterOn, AMK_bDcOn, AMK_bEnable, AMK_bErrorReset)

AMK_bDcOn_shift = bitsll(uint8(AMK_bDcOn),1);               %shift DcOn bit 1 times to left
AMK_bEnable_shift = bitsll(uint8(AMK_bEnable),2);           %shift Enable bit 2 times to left
AMK_bErrorReset_shift = bitsll(uint8(AMK_bErrorReset),3);   %shift ErrorReset bit 3 times to left

AMK_Control = uint8(AMK_bInverterOn);                           %bit 0 is InvertOn bit
AMK_Control = bitor(AMK_Control,uint8(AMK_bDcOn_shift));        %bitwise OR AMK_Control with shifter DcOn bit
AMK_Control = bitor(AMK_Control,uint8(AMK_bEnable_shift));      %bitwise OR AMK_Control with shifted Enable bit
AMK_Control = bitor(AMK_Control,uint8(AMK_bErrorReset_shift));  %bitwise OR AMK_Control with shifted ErrorReset bit

== matlab function rti1401_program_controls_2018/Processor/Bypass/Torque Vectoring Bypass ==
  data: torqueBypass output; sensors input; rpmBypass output; car parameter
function [torqueBypass,rpmBypass]= TV_Bypass(sensors, car)

PmaxTyre = car.Pmax_bypass*0.25; %max bypass power divided over wheels
TmaxTyre = PmaxTyre./max(sensors.wheelspeed,1); %transformation with highest wheel speed
TmaxMotor= TmaxTyre*car.gearRatio;
powercheck = 0.8;%sum(TmaxMotor)/sum(car.motor.Tmax);

torqueBypass = (car.motor.Tmax*(sensors.throttle/100)*...
    powercheck).*[0.666;0.666;1;1]; %basic 0.4/0.6 distirbution

if sensors.throttle > 0
    rpmBypass = car.motor.rpmMax;
else
    rpmBypass = [0;0;0;0];
end

%torqueBypass = max(min(torqueBypass,TmaxTyre),-TmaxTyre); %implausibility check

== matlab function rti1401_program_controls_2018/Processor/Control Systems/Distributor/MATLAB Function ==
  data: sensors input; torqueDistribution output; settings input; estimPar input; car parameter; Mz input; slipSet output; Fdes output; Fxmax output; Fx output; Fdes input
function [torqueDistribution, slipSet,Fdes,Fxmax, Fx]= TorqueDistributor(sensors,settings, estimPar, car, Mz, Fdes)
%,Fdes,sumFx,Fxmax,Fxmaxsum

torqueDistribution = [0;0;0;0];
slipSet = [0;0;0;0];


sumFx=0;
Fxmax=[0;0;0;0];
Fxmaxsum=0;
Fx=[0;0;0;0];
if settings.torqueMode == 1
    
    dT =  0.25*Mz/(car.tw*0.5)*car.tireRadius;
    torqueDistribution = car.motor.Tmax*sensors.throttle;
    torqueDistribution = torqueDistribution + [-1; 1; -1; 1]*dT;
    
    for i=1:4
        if torqueDistribution(i) > 0
            slipSet(i) = car.TC.slipSetAcc;
        else
            slipSet(i) = car.TC.slipSetBrake;
        end
    end
    
    
end



%Test torque mode: only Fx, no steeringAngle

if settings.torqueMode == 2
    

    
    Fxmax = [0;0;0;0];
    %minForce = 2*car.Cd*car.AFront*0.5*car.rhoAir*estimPar.v*estimPar.v*0.25; %2* of niet? en met Cd?
    minForce = 0;
    FyReduceFactor = 0.1;
    Fxmax = max((estimPar.mu .* estimPar.Fzi).^2-FyReduceFactor*estimPar.Fyi.^2,0).^0.5; %Kamm's circle
    %Fxmax = estimPar.mu.*estimPar.Fzi;
    
    Fxmax = max(Fxmax,minForce);
    
    FxmaxMax = car.gearRatio*car.motor.Tmax/car.tireRadius; %make sure the max torque of the motor isn't surpassed
    checkFxmax = find((Fxmax > FxmaxMax)==1);
    Fxmax(checkFxmax)=FxmaxMax(checkFxmax);
    
    if settings.unlimitedFx == 1  %Surpass the tyre grip limits in case if the driver feels to restricted with this.
        Fxmax = FxmaxMax;
    end
    
    Fxmaxsum = sum(Fxmax);
    Fxmin = -Fxmax*settings.Regen;
    
    Fx = [0;0;0;0];
    
    
    Fx = Distributor(settings, car, Mz, Fdes, Fxmax, Fxmin);
    
    torqueDistribution = car.tireRadius*Fx; %torque of motor, NOT of wheels (as IPG expects this as input)
    
    for i=1:4
        if torqueDistribution(i) > 0
            slipSet(i) = car.TC.slipSetAcc;
        else
            slipSet(i) = car.TC.slipSetBrake;
        end
    end
    
    sumFx = sum(Fx);
end


end

== matlab function rti1401_program_controls_2018/Processor/Control Systems/Distributor/Torque//Brake analyzer/MATLAB Function1 ==
  data: sensors input; Fdes output; settings input; estimPar input; car parameter; aero input
function Fdes = Fdes(sensors, settings, estimPar, car, aero)
    
    Fdes = sum(sensors.throttle*1.5*estimPar.mu*(car.mass*car.g + aero.FL))*car.gearRatio;
    
    if sensors.brake > 0
        Fdes = -sum(car.motor.Tmax)*sensors.brake/car.tireRadius*car.gearRatio;
    end   

end

== matlab function rti1401_program_controls_2018/Processor/Control Systems/Power Checker/Power checker ==
  data: sensors input; settings input; estimPar input; UncheckedTorque input; CheckedTorque output; car parameter
function CheckedTorque = fcn(sensors,settings,estimPar, UncheckedTorque,car)

%% Power limiter according to FS rules

P_mech = sum(UncheckedTorque.*sensors.wheelspeed*car.gearRatio); %[Nm*rad/s][W]

maxMechPower = (car.Pmax - car.PC.safetyMargin)*estimPar.eff;
power2beReduced = 0;

if P_mech > maxMechPower
    power2beReduced = P_mech - maxMechPower;
end

if abs(P_mech) > 0.1
    part2beReduced = power2beReduced/P_mech;
else
    part2beReduced = 0;
end

CheckedTorque = UncheckedTorque*max(min((1 - part2beReduced),1),0);
CheckedP_mech = sum(CheckedTorque.*sensors.wheelspeed*car.gearRatio); %[Nm*rad/s][W]

== matlab function rti1401_program_controls_2018/Processor/Vehicle Estimated Parameters/Wheel speed calculation ==
  data: sensors input; beta_lin input; y_meas output; car parameter
function y_meas  = wheelspeedcalc(sensors, beta_lin, car)

yaw_rate = sensors.yawRate;
ay = sensors.accy;
vxfl = sensors.wheelspeed(1)*car.tireRadius;
vxfr = sensors.wheelspeed(2)*car.tireRadius;
vxrl = sensors.wheelspeed(3)*car.tireRadius;
vxrr = sensors.wheelspeed(4)*car.tireRadius;

y_meas = [yaw_rate ay vxfl vxfr vxrl vxrr beta_lin];

== matlab function rti1401_program_controls_2018/Processor/Vehicle Estimated Parameters/Global model calculation ==
  data: sensors input; F_KF output; States input; H_KF output; y_pred output; yawrate_lin output; beta_lin output; car parameter
function [F_KF, H_KF, y_pred, yawrate_lin, beta_lin] = global_model(sensors, States, car)

global vy_g psi_dot_g vx_g Cf_g Cr_g vy_lin psi_dot_lin

if isempty(vy_g) == 1 && isempty(psi_dot_g) == 1 && isempty(vx_g) == 1 ...
        && isempty(Cf_g) == 1 && isempty(Cr_g) == 1 
    States.vy_g = 0;
    States.psi_dot_g = 0;
    States.vx_g = 0;
    States.Cf_g = 0;
    States.Cr_g = 0;
    
else 
    
    States.vy_g = vy_g;
    States.psi_dot_g = psi_dot_g;
    States.vx_g = vx_g;
    States.Cf_g = Cf_g;
    States.Cr_g = Cr_g;
    delta = (sensors.wheelAngles(1)+sensors.wheelAngles(2))/2;
    
    %% Calculating F_KF %%
    
    F_vy = [-(2*(States.Cf_g+States.Cr_g))/(car.mass*States.vx_g),...
        -((2*(States.Cf_g*car.lf-States.Cr_g*car.lr))/(car.mass*States.vx_g))+States.vx_g,...
        (((2*(States.Cf_g+States.Cr_g))/(car.mass*States.vx_g^2))*States.vy_g)+...
        (((2*(States.Cf_g*car.lf-States.Cr_g*car.lr))/(car.mass*States.vx_g^2))*States.psi_dot_g)-States.psi_dot_g,...
        (-2/(car.mass*States.vx_g))*(States.vy_g+car.lf*States.psi_dot_g)+(2*delta/car.mass),...
        (-2/(car.mass*States.vx_g))*(States.vy_g-car.lr*States.psi_dot_g)];
    
    F_psi_dot = [-(2*(States.Cf_g*car.lf-States.Cr_g*car.lr))/(car.yawInertia*States.vx_g),...
        -((2*(States.Cf_g*car.lf^2+States.Cr_g*car.lr^2))/(car.yawInertia*States.vx_g)),...
        (((2*(States.Cf_g*car.lf-States.Cr_g*car.lr))/(car.yawInertia*States.vx_g^2))*States.vy_g)+...
        (((2*(States.Cf_g*car.lf^2+States.Cr_g*car.lr^2))/(car.yawInertia*States.vx_g^2))*States.psi_dot_g),...
        (-2*car.lf/(car.yawInertia*States.vx_g))*(States.vy_g+car.lf*States.psi_dot_g)+(2*delta*car.lf/car.yawInertia),...
        (2*car.lr/(car.yawInertia*States.vx_g))*(States.vy_g-car.lr*States.psi_dot_g)];
    
    F_vx = [States.psi_dot_g, States.vy_g,0,0,0];
    
    F_Cf = [0,0,0,0,0];
    
    F_Cr = [0,0,0,0,0];
    
    F_KF = [F_vy;F_psi_dot;F_vx;F_Cf;F_Cr];
    
    %% Calculation vy_lin and beta_lin %% Gelineariseerd, hier kan eventueel ook
    % ode45 voor gebruikt worden.
    
   A_1 = (-2*(car.Cf_lin + car.Cr_lin))/(car.mass*States.vx_g);
   A_2 = -((2*(car.Cf_lin*car.lf - car.Cr_lin*car.lr))/(car.mass*States.vx_g))+States.vx_g;
   A_3 = -(2*(car.Cf_lin*car.lf - car.Cr_lin*car.lr))/(car.yawInertia*States.vx_g);
   A_4 = (-2*(car.Cf_lin*car.lf^2 + car.Cr_lin*car.lr^2))/(car.yawInertia*States.vx_g);
   
   B_1 = (2*car.Cf_lin*delta)/(car.mass);
   B_2 = (2*car.Cf_lin*car.lf*delta)/(car.yawInertia);
      
   A = [1+A_1*car.dt, A_2*car.dt; A_3*car.dt 1+A_4*car.dt];
   B = [B_1; B_2];
   
   
   lin_var = A*[vy_lin;psi_dot_lin] + B;
   vy_lin = lin_var(1);
   psi_dot_lin = lin_var(2);
   yawrate_lin =  psi_dot_lin;
   beta_lin = vy_lin/(States.vx);
    
    %% Calculation H_KF %%
    
    H_psi_dot = [0, 1, 0, 0,0];
    
    H_ay = [-(2*(States.Cf_g+States.Cr_g))/(car.mass*States.vx_g),...
        -((2*(States.Cf_g*car.lf-States.Cr_g*car.lr))/(car.mass*States.vx_g)),...
        (((2*(States.Cf_g+States.Cr_g))/(car.mass*States.vx_g^2))*States.vy_g)+...
        (((2*(States.Cf_g*car.lf-States.Cr_g*car.lr))/(car.mass*States.vx_g^2))*States.psi_dot_g),...
        (-2/(car.mass*States.vx_g))*(States.vy_g+car.lf*States.psi_dot_g)+(2*delta/car.mass),...
        (-2/(car.mass*States.vx_g))*(States.vy_g-car.lr*States.psi_dot_g)];
    
    H_vxfl = [sin(sensors.wheelAngles(1)),  -(car.tf/2)*cos(sensors.wheelAngles(1))+car.lf*sin(sensors.wheelAngles(1)), cos(sensors.wheelAngles(1)), 0, 0];
    
    H_vxfr = [sin(sensors.wheelAngles(2)), (car.tf/2)*cos(sensors.wheelAngles(2))+car.lf*sin(sensors.wheelAngles(2)), cos(sensors.wheelAngles(2)),  0, 0];
    
    H_vxrl = [0, -(car.tr/2), 1, 0, 0];
    
    H_vxrr = [0, (car.tr/2), 1, 0, 0];
    
    H_beta_lin = [0,0,-(vy_lin/States.vx_g^2),0,0]; %afgeleide naar vx herplaatst, die naar vy = 0?
    
    H_KF = [H_psi_dot;H_ay;H_vxfl;H_vxfr;H_vxrl;H_vxrr; H_beta_lin];

    %% Calculation of y_pred
    
    y_pred.yawrate = States.psi_dot_g;
    
    y_pred.ay = (-2*(States.Cf_g+States.Cr_g)/(car.mass*States.vx_g))*(States.vy) - ...
        (2*(States.Cf_g*car.lf-States.Cr_g*car.lr)/(car.mass*States.vx_g))*(States.psi_dot_g) +... % - teken aangepast naar vgl (7) uit van Aalst
        (2*States.Cf_g*delta/car.mass);
    
    y_pred.vxfl = (States.vx_g - States.psi_dot_g*(car.tf/2))*cos(sensors.wheelAngles(1)) + ...
        (States.vy_g + States.psi_dot_g*(car.lf/2))*sin(sensors.wheelAngles(1));
    
    y_pred.vxfr = (States.vx_g + States.psi_dot_g*(car.tf/2))*cos(sensors.wheelAngles(2)) + ...
        (States.vy_g + States.psi_dot_g*(car.lf/2))*sin(sensors.wheelAngles(2));
    
    y_pred.vxrl = (States.vx_g - States.psi_dot_g*(car.tr/2));
    
    y_pred.vxrr = (States.vx_g + States.psi_dot_g*(car.tr/2));
    
    y_pred.beta_lin = (vy_lin)/(States.vx);
    
end
end

== matlab function rti1401_program_controls_2018/Processor/Control Systems/Traction Control ==
  data: sensors input; Torques output; settings input; estimPar input; torqueDistribution input; slipSet input; car parameter; TiTi2 output; error output; rpmSet output
function [Torques, TiTi2, error, rpmSet] = Traction(sensors, settings, estimPar, torqueDistribution, slipSet, car)

error =[0 0 0 0]';
persistent errorInt; if isempty(errorInt); errorInt=[0 0 0 0]'; end
persistent errorD; if isempty(errorD); errorD=[0 0 0 0]'; end
persistent errorPrev; if isempty(errorPrev); errorPrev=[0 0 0 0]'; end

%persistent wi_prev; if isempty(wi_prev); wi_prev=[0 0 0 0]'; end
%persistent SR_expected; if isempty(SR_expected); SR_expected=zeros(4, 8); end
%persistent wvi_prev; if isempty(wvi_prev); wvi_prev=[0 0 0 0]'; end

persistent TiPrev; if isempty(TiPrev); TiPrev=[0 0 0 0]'; end

persistent errorInt2; if isempty(errorInt2); errorInt2=[0 0 0 0]'; end
persistent Ti; if isempty(Ti); Ti=[0 0 0 0]'; end
persistent Ti2; if isempty(Ti2); Ti2=[0 0 0 0]'; end

rpmSet = [20000;20000;20000;20000];

if settings.TC == 1

    slipRatioTarget = slipSet;
    dist = estimPar.Fzi/sum(estimPar.Fzi);
    
    Kp = 100*dist*10;
    Ki = 40*dist*1000;
    Kd = 0*dist/100;
    Kv = 70/100;
    Mu = car.mu;
    
    Kp2 = 20*dist/1000;
    Ki2 = 40*dist/1000;
    
    %normal non linear torque control
    error = slipRatioTarget - estimPar.slip;
    
    errorInt = errorInt + error*car.dt;
    errorInt = min(max(errorInt,-0.001*[1;1;1;1]),0.003*[1;1;1;1]);
    errorD = min(max(errorD*0.1 + 0.9*(error - errorPrev)/car.dt,-25),25);
    lambdaD = Kp.*error + Ki.*errorInt + Kd.*errorD;
    Ti = lambdaD*car.tireInertia*max(estimPar.v,0)^Kv/car.tireRadius + sign(torqueDistribution).*estimPar.Fzi*(Mu)*car.tireRadius;
    Ti = Ti / car.gearRatio;
    
    %optimum seeking
    dFds = dFdsCalculator(estimPar.Fxi,estimPar.slip);
    error2 = dFds - 0;
    errorInt2 = errorInt2 + error2*car.dt;
    errorInt2 = min(max(errorInt2,-500*[1;1;1;1]),500*[1;1;1;1]);
    lambdaD2 = Kp2.*error2 + Ki2.*errorInt2;
    Ti2 = lambdaD2*car.tireInertia*max(estimPar.v,0)^Kv/car.tireRadius + sign(torqueDistribution).*estimPar.Fzi*(car.TC_mu)*car.tireRadius;
    Ti2 = Ti2 / car.gearRatio;
    
    for i=1:4
        if abs(error(i)) < 0.05
            Ti(i) = Ti2(i);
        end
    end
    
    if estimPar.v < 1/3.6
        %Ti = [80 80 180 180]';
        errorInt = [0 0 0 0]';
    end

    if sensors.throttle < 0.1
        errorInt = [0 0 0 0]';
    end
    
    lowerBoundary = TiPrev - 100/car.gearRatio;
    upperBoundary = TiPrev + 100/car.gearRatio;

    Ti = min(max(Ti,lowerBoundary),upperBoundary);
    
    TiPrev = Ti;
    errorPrev = error;
    
    Torques = Ti;
    for i=1:4
        if torqueDistribution(i) > 0
            Torques(i) = max(min(Torques(i),torqueDistribution(i)),0); 
        else
            Torques(i) = min(max(Torques(i),torqueDistribution(i)),0);
        end
    end
    
    
else
    Torques = torqueDistribution;
end

checkTorquemax = find((Torques > car.motor.Tmax)==1); %Limit torques to max torque
Torques(checkTorquemax)=car.motor.Tmax(checkTorquemax);



%wi_prev = sensors.wheelspeed;
%wvi_prev = sensors.wheelspeedi;

TiTi2 = [Ti;Ti2];

end

function [dFds] = dFdsCalculator(Fx,slipRatio)
N = 6;

persistent slipVector, if isempty(slipVector); slipVector = zeros(N,4); end
persistent FxVector, if isempty(FxVector); FxVector = zeros(N,4); end


FxVector(1,:) = Fx;
slipVector(1,:) = slipRatio;

dFds = [0;0;0;0];

for i=1:4
    p1 = polyfit(slipVector(:,i),FxVector(:,i),1);
    p2 = polyfit(FxVector(:,i),slipVector(:,i),1);
    
    rico1 = p1(1);
    rico2 = 1/p2(1);
    
    rico = sign(min(abs(rico1),abs(rico2)))*min(abs(rico1),abs(rico2));

    dFds(i) = max(min(rico,20000),-20000);
end

% shift list one
dummy = FxVector(1:N-1,:);
FxVector = [[0,0,0,0];dummy];
dummy = slipVector(1:N-1,:);
slipVector = [[0,0,0,0];dummy];

end
